simulink library "PowerFlowLib"  (R2016a)
settings: Solver=ode45  StartTime=0.0  StopTime=10.0  RelTol=1e-3
undefined symbols (not defined in the file or in its folder): Air, AirProp, C, F1, F2, Fanmap, Fld1, Fld2, Fluid, fueltankdata, HydProp, HydraulicLoad, IBFD_exc, L, LoadFluidProps, magnitude, MSSN, n_alghts, PumpProp, pwr_alghts, R_fd_exc, Rcore, Ts, VBFD_exc
libraries: PowerFlowLib x35, simulink x19, powerlib_extras x2, dspstat3 x2
(part 5 of 12)

== system PowerFlowLib/Energy & Power Systems/Electrical/Machines ==
  note: Electric Machines
  DC Position Servo : Subsystem  mask{Vf=390, Ra=0.5, La=0.9e-3, Rfsh=400, Lfsh=320, Lmsh=1.9, J=1.5, Ki=0.1}
      mask prompts: Vf "Field voltage (V)"; Ra "Armature resistance (Ohms)"; La "Armature inductance (H)"; Rfsh "Shunt field resistance (Ohms)"; Lfsh "Shunt field inductance (H)"; Lmsh "Mutual inductance (H)"; J "Rotor moment of inertia (Kgm^2)"; Ki "Integral constant for position loop (Ki)"
  DC Speed Servo : Subsystem  mask{Vf=390, Ra=0.05, La=0.9e-3, Rfsh=400, Lfsh=320, Lmsh=1.9, J=1.5}
      mask prompts: Vf "Field voltage (V)"; Ra "Armature resistance (Ohms)"; La "Armature inductance (H)"; Rfsh "Shunt field resistance (Ohms)"; Lfsh "Shunt field inductance (H)"; Lmsh "Mutual inductance (H)"; J "Rotor moment of inertia (Kgm^2)"
  Induction motor : Subsystem
      mask help: Induction Motor Model.
      mask init:
      | IM_fan_omega=[0;52.36;104.72;157.08;188.50;209.44;261.80;314.16;366.52;...
      |       376.99;418.88;471.24;523.60;565.49;575.96;628.32;680.68;733.04];
      | IM_fan_torque=[0;0.363;0.561;0.603;0.614;0.621;0.683;0.868;0.950;0.992;...
      |       1.134;1.269;1.460;1.700;1.750;2.044;2.262;2.618];
      |   
      | IM_wb=2*pi*200;  %base frequency
      | V_rated=132.8;  %rated phase voltage
      | IM_Lpr=114e-6; %Referred rotor leakage inductance
      | IM_Ls=114e-6;  %Stator leakage inductance
      | IM_Lm=0.0036;  %Magnetizing inductance
      | IM_rs=.0248; %Stator series resistance
      | IM_rrp=.01438; %referred rotor series resistance
      | IM_Xplr=IM_wb*IM_Lpr; %referred rotor leakage reactance
      | IM_Xls=IM_wb*IM_Ls;  %stator leakage reactance
      | IM_Xm=IM_wb*IM_Lm; %Magnetizing reactance
      | 
      | IM_Xr=IM_Xm+IM_Xplr;
      | IM_Xs=IM_Xm+IM_Xls;
      | IM_XM=1/(1/IM_Xm+1/IM_Xls+1/IM_Xplr);
      | IM_Lsp=1/IM_wb*(IM_Xls-IM_Xm^2/IM_Xplr);
      | IM_LR = IM_Lpr+IM_Lm;
      | IM_LS = IM_Ls+IM_Lm;
      | 
      | IM_Poles = 4;
      mask Display:
      | p1 = 0:0.1:(2*pi+0.1);
      | plot(sin(p1), cos(p1));
      | plot(0.8*sin(p1), 0.8*cos(p1));
      | plot(0.7*sin(p1), 0.7*cos(p1));
      | plot(0.3*sin(p1), 0.3*cos(p1));
      | p2 = 0:(pi/8):(2*pi);
      | for i = 1:length(p2);
      |     plot(0.05*sin(p1)+0.6*sin(p2(i)), 0.05*cos(p1)+0.6*cos(p2(i)));
      | end
      | port_label('output',1,'T_em')
      | port_label('output',2,'iqs')
      | port_label('output',3,'ids')
      | port_label('output',4,'i0s')
      | port_label('input',1,'vqs')
      | port_label('input',2,'vds')
      | port_label('input',3,'v0s')
      | port_label('input',4,'wr_mech')
  Permanent Magnet Synchronous Generator1 : Subsystem
      mask help: Permanent Magnet Synchronous Machine Model.
      mask init:
      | data_PMSM = load('exciter.mat');
      |   
      | % Lls_pm=500e-6;
      | % Lq=1.6e-3+Lls_pm;
      | % Ld=1e-3+Lls_pm;
      | Lls_pm = 5e-3;
      | Ld = data_PMSM.r(2);
      | Lq = data_PMSM.r(3);
      | Jm=data_PMSM.r(6);
      | l_m=data_PMSM.r(4);
      | Rs_pm=data_PMSM.r(1);
      | Poles = data_PMSM.r(5);
      | R_conv_exciter = 1/data_PMSM.r(7);
      | mc_exciter = data_PMSM.r(8);
      mask Display:
      | p1 = 0:0.1:(2*pi+0.1);
      | plot(sin(p1), cos(p1));
      | plot(0.8*sin(p1), 0.8*cos(p1));
      | plot(0.7*sin(p1), 0.7*cos(p1));
      | plot(0.3*sin(p1), 0.3*cos(p1));
      | plot([-0.2 0.2], [0.4 0.4], [0.2 0.3], [0.4 0.5], [-0.3 -0.2], [0.5 0.4]);
      | plot([-0.1 0.1], [0.6 0.6], [-0.1 0.1], [-0.6 -0.6], [0.6 0.6], [-0.1 0.1], [-0.6 -0.6], [-0.1 0.1]);
      | plot([0.4 0.4], [0.2 -0.2], [0.4 0.5], [0.2 0.3], [0.4 0.5], [-0.2 -0.3]);
      | plot([-0.2 0.2], [-0.4 -0.4], [0.2 0.3], [-0.4 -0.5], [-0.3 -0.2], [-0.5 -0.4]);
      | plot([-0.4 -0.4], [0.2 -0.2], [-0.4 -0.5], [0.2 0.3], [-0.4 -0.5], [-0.2 -0.3]);
      | port_label('output',1,'vqd0')
      | port_label('output',2,'Te')
      | port_label('output', 3, 'Ploss');
      | port_label('input',1,'iqd0')
      | port_label('input',2,'wr_m')
  Synchronous Machine P.U. dq0 : Subsystem  mask{machine_mode=20kVA_Gen}
      mask prompts: machine_mode "Machine Preset"
      mask help: Synchronous Machine p.u. Model in dq0 Frame.
      mask init:
      | switch machine_mode
      |     case 1
      |         preset = '20kVA_Gen.mat';
      |     case 2
      |         preset = '52.5kVA_Gen.mat';
      |     case 3
      |         preset = '100kVA_Gen.mat';
      |     case 4
      |         preset = '300kVA_Gen.mat';
      |     case 5
      |         preset = '800kVA_Gen.mat';
      |     otherwise
      |         preset = '1MVA_Gen.mat';
      | end
      | 
      | data = load(preset);
      | 
      | % Stator
      | Rs = data.r(1);
      | Xls = data.r(2);
      | Xmd = data.r(3);
      | Xmq = data.r(4);
      | 
      | % Field
      | R_fd = data.r(5);
      | Xlfd = data.r(6);
      | % Dampers
      | R_1d = data.r(7);
      | Xl1d = data.r(8);
      | R_1q = data.r(9);
      | Xl1q = data.r(10);
      | R_2q = data.r(11);
      | Xl2q = data.r(12);
      | 
      | % Rotor
      | P = data.r(13);
      | ws = data.r(14);
      | 
      | % Inductances
      | Xd = Xls + Xmd;
      | Xq = Xls + Xmq;
      | Xfd = Xlfd + Xmd;
      | X1q = Xl1q + Xmq;
      | Xd1 = Xd - Xmd^2/Xfd;
      | Xq1 = Xq - Xmq^2/X1q;
      | Xd2 = Xls + (1/(1/Xmd + 1/Xlfd + 1/Xl1d));
      | Xq2 = Xls + (1/(1/Xmq + 1/Xl1q + 1/Xl2q));
      | Tdo1 = Xfd/ws/R_fd;
      | Tqo1 = X1q/ws/R_1q;
      | Tdo2 = 1/ws/R_1d*(Xl1d + 1/(1/Xmd + 1/Xlfd));
      | Tqo2 = 1/ws/R_2q*(Xl2q+1/(1/Xmq + 1/Xl1q));
      | 
      | % Transmission Line
      | RTL = data.r(15);
      | XTL = data.r(16);
      | 
      | % Regulator and Governor
      | KA = data.r(17);
      | KF = data.r(18);
      | T_f = data.r(19);
      | TA = data.r(20);
      | KE = data.r(21);
      | TE = data.r(22);
      | 
      | % Base Quantities
      | SB = data.r(23);
      | VBDQ = data.r(24);
      | wB = data.r(25);
      | P = data.r(13);
      | H = data.r(26);
      | 
      | TB = (P/2)*SB/wB;
      | IBDQ = SB/VBDQ;
      | LBDQ = VBDQ/wB;
      | 
      | IBFD = IBDQ;
      | IB1D = IBDQ;
      | IB1Q = IBDQ;
      | IB2Q = IBDQ;
      | 
      | VBFD = SB/IBFD;
      | VB1D = SB/IB1D;
      | VB1Q = SB/IB1Q;
      | VB2Q = SB/IB2Q;
      | 
      | LBFD = VBFD/wB;
      | LB1D = VB1D/wB;
      | LB1Q = VB1Q/wB;
      | LB2Q = VB2Q/wB;
      | 
      | J = 2*data.r(26)/(wB*2/P)^2*SB;
      | M = 2*H/wB;
      | 
      | R_conv_gen = 1/data.r(27);
      | mc_gen = data.r(28);
      mask TypeOptions machine_mode: 20kVA_Gen | 52.5kVA_Gen | 100kVA_Gen | 300kVA_Gen | 800kVA_Gen | 1MVA_Gen
      mask Display:
      | p = 0:0.1:(2*pi+0.1);
      | plot(sin(p), cos(p));
      | p1 = (-pi/8-0.1-0.2):0.1:(pi/8+0.1-0.2);
      | plot(0.8*sin(p1), 0.8*cos(p1), 0.8*sin(p1+pi), 0.8*cos(p1+pi));
      | p2 = sin((-pi/8-0.1-0.2+pi/8+0.1-0.2)/2);
      | p3 = sin((-pi/8-0.1-0.2+pi/8+0.1-0.2)/2+pi);
      | p4 = cos((-pi/8-0.1-0.2+pi/8+0.1-0.2)/2);
      | p5 = cos((-pi/8-0.1-0.2+pi/8+0.1-0.2)/2+pi);
      | plot(0.8*[p2, p3], 0.8*[p4, p5]);
      | port_label('output', 1, 'Vdq0');
      | port_label('output', 2, 'Te');
      | port_label('output', 3, 'Vfd');
      | port_label('output', 4, 'Ploss');
      | port_label('input', 1, 'idq0');
      | port_label('input', 2, 'w');
      | port_label('input', 3, 'ifd');
  Transformer : Subsystem  mask(Transformer){Rp=0.005, Rs=0.1, N1=32, N2=355}
      mask prompts: Rp "Primary Winding Resistance"; Rs "Secondary Winding Resistance"; N1 "Number of Turns in Primary"; N2 "Number of Turns in Secondary"
      mask help:
      | The user inputs and outputs are given below. Inputs to the model are:
      |
      | Block Inputs
      | #1: Primary voltage input [V]
      | #2: Secondary current input [A]
      |
      | Block Outputs
      | #1: Secondary voltage output [V]
      | #2: Primary current input [A]
      mask Help: eval('open(''Transformer Help.html'')');
      mask Display:
      | image(imread('Transformer.png'))
      | 
      | port_label('input',1,'{\bf V_i_n}','TexMode','on')
      | port_label('input',2,'{\bf I_o_u_t}','TexMode','on')
      | 
      | port_label('output',1,'{\bf V_o_u_t}','TexMode','on')
      | port_label('output',2,'{\bf I_i_n}','TexMode','on')

== system PowerFlowLib/Energy & Power Systems/Electrical/Rectifiers ==
  note: Rectifier
  Single-phase Full Bridge Practical : Subsystem  mask(Single-phase full bridge rectifier.){C=100e-6, Rc=1}
      mask prompts: C "Output capacitance (F):"; Rc "Circuit parasitic resistance (ohm):"
      mask help: Single-phase Full bridge rectifier. Lead resistance is added to make simulation possible.
  Single-phase Half Bridge : Subsystem  mask(Single-phase half bridge rectifier.){C=100e-6, Rc=1}
      mask prompts: C "Output capacitance (F):"; Rc "Circuit parasitic resistance (ohm):"
      mask help: Single-phase half bridge rectifier. Lead resistance is added to make simulation possible.
  Three Phase Full Bridge Practical : Subsystem  mask(Single-phase full bridge rectifier.){C=100e-6, Rc=1}
      mask prompts: C "Output capacitance (F):"; Rc "Circuit parasitic resistance (ohm):"
      mask help: Single-phase Full bridge rectifier. Lead resistance is added to make simulation possible.
  Three-phase Full Bridge1 : Subsystem  mask(Single-phase full bridge rectifier.){C=100e-6, Rc=1}
      mask prompts: C "Output capacitance (F):"; Rc "Circuit parasitic resistance (ohm):"
      mask help: Single-phase Full bridge rectifier. Lead resistance is added to make simulation possible.
  three-phase active rectifier : Subsystem
      mask help: 3 phase active rectifier
  three-phase active rectifier Voltage Mode : Subsystem  mask(Rectifier){L=1e-3, C=1e-4}
      mask prompts: L "Inductance"; C "Capacitance"
      mask help:
      | The rectifier block converts ac voltage to dc voltage, which interfaces with the rest of the DC system.
      | This is an active rectifier and it is modeled in the synchronous dq0 reference frame.
      | The active rectifier control algorithm is omitted and a simplified model is implemented.
      |
      | Block Inputs:
      |
      | #1: Input line voltage in the synchronous reference frame [V]
      | #2: Converter modulation depth. It is a number between 0 and 1
      | #3: Output dc voltage level [V]
      |
      | Block Outputs:
      |
      | #1: Output DC current level [A]
      | #2: Input line current in the synchronous reference frame  [A]
      mask Display:
      | image(imread('Rectifier.png'))
      | 
      | % Define inputs
      | 
      | port_label('input',1,'{\bf V_d_q_0}','Texmode','on')
      | port_label('input',2,'{\bf m}','Texmode','on')
      | port_label('input',3,'{\bf V_D_C}','Texmode','on')
      | 
      | % Define outputs
      | 
      | port_label('output',1,'{\bf I_D_C}','Texmode','on')
      | port_label('output',2,'{\bf I_d_q_0}','Texmode','on')

== system PowerFlowLib/Energy & Power Systems/Electrical/Systems ==
  2 stage Boost converter (CCM Steady State) : Subsystem  mask(Cascaded Boost Converter CCM){KP=5, KI=1, VREF1=120}
      mask prompts: KP "Proportional constant"; KI "Integral constant"; VREF1 "Enter Stage 1 reference voltage (V) (Between 100 V and 150 V)"
      mask help: Two stage Boost Converter operated in steady state with a PI controller for duty ratio
  AC Service Bus : Subsystem
      mask help: Service Bus Structure.
      mask Display:
      | image(imread('ACbus.png')) % Load image
      | 
      | % Define inputs
      | 
      | port_label('input',1,'{\bf Select}','Texmode','on')
      | port_label('input',2,'{\bf Supply #1}','Texmode','on')
      | port_label('input',3,'{\bf Supply #2}','Texmode','on')
      | port_label('input',4,'{\bf Load}','Texmode','on')
      | 
      | % Define outputs
      | 
      | port_label('output',1,'{\bf Bus Voltage}','Texmode','on')
      | port_label('output',2,'{\bf Supply #1 Current}','Texmode','on')
      | port_label('output',3,'{\bf Supply #2 Current}','Texmode','on')
  DC Service Bus : Subsystem  mask(DC Service Bus){}
      mask help: Service Bus
      mask Display:
      | image(imread('DCbus.png')) % Load image
      | 
      | % Define inputs
      | 
      | port_label('input',1,'{\bf Select}','Texmode','on')
      | port_label('input',2,'{\bf Supply #1}','Texmode','on')
      | port_label('input',3,'{\bf Supply #2}','Texmode','on')
      | port_label('input',4,'{\bf Load}','Texmode','on')
      | port_label('input',5,'{\bf Charge}','Texmode','on')
      | 
      | % Define outputs
      | 
      | port_label('output',1,'{\bf Bus Voltage}','Texmode','on')
      | port_label('output',2,'{\bf Supply #1 Current}','Texmode','on')
      | port_label('output',3,'{\bf Supply #2 Current}','Texmode','on')
  GND Service Bus : Subsystem
      mask help: Ground Supply.
      mask Display:
      | image(imread('GPU2.jpg')) % Load image
      | 
      | % Define inputs
      | 
      | port_label('input',1,'{\bf I_d_q_0}','Texmode','on')
      | 
      | % Define outputs
      | 
      | port_label('output',1,'{\bf V_d_q_0}','Texmode','on')
  Gearbox : Subsystem  mask(Gearbox){Gear_Ratio=0.5620, Gear_Efficiency=98}
      mask prompts: Gear_Ratio "Gear Ratio"; Gear_Efficiency "Efficiency [%]"
      mask help:
      | Captures the effect of gear ratio on output shaft speed and torque.
      |
      | Input 1: Speed input [RPM]
      | Input 2: Torque input [Nm]
      |
      | Output 1: Speed output [RPM]
      | Output 2: Torque output [Nm]
      |
      | To simulate multiple gear ratios, vector inputs can be used for Gear Ratio and Efficiency.  Block outputs will be vectored signals of the same order.
      | Speed output = Speed input x Gear Ratio
      mask Display:
      | image(imread('Gearbox.png')) % Load image
      | 
      | % Define inputs
      | 
      | port_label('input',1,'{\bf \omega_e_n_g}','Texmode','on')
      | port_label('input',2,'{\bf \tau_e_n_g}','Texmode','on')
      | 
      | % Define outputs
      | 
      | port_label('output',1,'{\bf \omega_s_h_a_f_t}','Texmode','on')
      | port_label('output',2,'{\bf \tau_s_h_a_f_t}','Texmode','on')
  Gen Bus w/ APU switch : Subsystem  mask{LOWVLIMIT=90, UPVLIMIT=250, bus_st=2}
      mask prompts: LOWVLIMIT "Low voltage limit for generator cut-off (V)"; UPVLIMIT "Upper voltage limit for generator cut-off (V)"; bus_st "Bus voltage monitoring interval (s)"
      mask help: Generator Bus Structure.
  Generation Unit Sync-Sync : Subsystem  mask{machine_mode=100kVA_Gen, Rs=0.0163, Xls=0.00054, Xmd=0.66176, Xmq=0.00099, R_fd=0.016, Xlfd=0.2092, R_1d=0.2047, Xl1d=0.6524, R_1q=0.0429, R_2q=0.0429, Xl1q=0.0639, Xl2q=0.0639, ws=377, RTL=0.001, XTL=0.1, KA=20, KF=0.063, T_f=0.35, TA=0.2, KE=1, TE=0.314, SB=100000, VBDQ=100, wB=377, P=6, H=0.1777, R_conv_gen=0.05, mc_gen=10000, Vnom=115, fan_load='init_fan_characteristics.mat', exciter_param='exciter.mat'}
      mask prompts: machine_mode "Machine Preset"; Rs "Stator Resistance [ohm]"; Xls "Stator Leakage Reactance [ohm]"; Xmd "Magnetizing Direct Axis Reactance [ohm]"; Xmq "Magnetizing Quadrature Axis Reactance [ohm]"; R_fd "Field Resistance [ohm]"; Xlfd "Field Leakage Reactance [ohm]"; R_1d "Transient Direct Axis Resistance [ohm]"; Xl1d "Transient Leakage Direct Axis Reactance [ohm]"; R_1q "Transient Quadrature Axis Resistance [ohm]"; R_2q "Subtransient Quadrature Axis Resistance [ohm]"; Xl1q "Transient Leakage Quadrature Axis Reactance [ohm]"; Xl2q "Subtransient Leakage Quadrature Axis Reactance [ohm]"; ws "Rotational Speed [rad/s]"; RTL "Resistance [ohm]"; XTL "Reactance [ohm]"; SB "Baes Complex Power [VA]"; VBDQ "Base Direct and Quadrature Axis Armature Voltage [V]"; wB "Base Electrical Frequency [rad/s]"; P "Number of Pole Pairs"; H "Shaft Inertia Constant [s]"; Vnom "Nominal Voltage [V]"; fan_load "Fan Load"; exciter_param "Exciter Machine Parameters"
      mask help:
      | A generator system block implements a generic power generation unit consisting of a gearbox, a synchronous generator, a synchronous exciter and exciter controls.
      | The generator size can be selected from the drop window below.
      | (For advanced-users) When the User-defined option is selected from the drop window, the generator parameters can be manually specified in the tabs below.
      |
      | Block Inputs:
      |
      | #1: Jet engine low pressure spool [RPM]
      | #2: Exciter system supply voltage [V]
      | #3: Synchronous reference frame line currents  [A]
      |
      | Block Output:
      |
      | #1: Synchronous reference frame line voltages [V]
      | #2: Exciter system supply current [A]
      | #3: Electromagnetic torque on the low pressure spool  [N-M]
      | #4: Heat rejected to the cooling system or ambient [W]
      mask init:
      | load(fan_load);
      | 
      | % Inductances
      | Xd = Xls + Xmd;
      | Xq = Xls + Xmq;
      | Xfd = Xlfd + Xmd;
      | X1q = Xl1q + Xmq;
      | Xd1 = Xd - Xmd^2/Xfd;
      | Xq1 = Xq - Xmq^2/X1q;
      | Xd2 = Xls + (1/(1/Xmd + 1/Xlfd + 1/Xl1d));
      | Xq2 = Xls + (1/(1/Xmq + 1/Xl1q + 1/Xl2q));
      | Tdo1 = Xfd/ws/R_fd;
      | Tqo1 = X1q/ws/R_1q;
      | Tdo2 = 1/ws/R_1d*(Xl1d + 1/(1/Xmd + 1/Xlfd));
      | Tqo2 = 1/ws/R_2q*(Xl2q+1/(1/Xmq + 1/Xl1q));
      | 
      | % Base Quantities
      | 
      | TB = (P/2)*SB/wB;
      | IBDQ = SB/VBDQ;
      | LBDQ = VBDQ/wB;
      | 
      | IBFD = IBDQ;
      | IB1D = IBDQ;
      | IB1Q = IBDQ;
      | IB2Q = IBDQ;
      | 
      | VBFD = SB/IBFD;
      | VB1D = SB/IB1D;
      | VB1Q = SB/IB1Q;
      | VB2Q = SB/IB2Q;
      | 
      | LBFD = VBFD/wB;
      | LB1D = VB1D/wB;
      | LB1Q = VB1Q/wB;
      | LB2Q = VB2Q/wB;
      | 
      | J = 2*H/(wB*2/P)^2*SB;
      | M = 2*H/wB;
      | 
      | % Exciter
      | 
      | data_exc = load(exciter_param);
      |   
      | % Stator
      | Rs_exc = data_exc.r(1);
      | Xls_exc = data_exc.r(2);
      | Xmd_exc = data_exc.r(3);
      | Xmq_exc = data_exc.r(4);
      | 
      | % Field
      | R_fd_exc = data_exc.r(5);
      | Xlfd_exc = data_exc.r(6);
      | % Dampers
      | R_1d_exc = data_exc.r(7);
      | Xl1d_exc = data_exc.r(8);
      | R_1q_exc = data_exc.r(9);
      | Xl1q_exc = data_exc.r(10);
      | R_2q_exc = data_exc.r(11);
      | Xl2q_exc = data_exc.r(12);
      | 
      | % Rotor
      | P_exc = data_exc.r(13);
      | ws_exc = data_exc.r(14);
      | 
      | % Inductances
      | Xd_exc = Xls_exc + Xmd_exc;
      | Xq_exc = Xls_exc + Xmq_exc;
      | Xfd_exc = Xlfd_exc + Xmd_exc;
      | X1q_exc = Xl1q_exc + Xmq_exc;
      | Xd1_exc = Xd_exc - Xmd_exc^2/Xfd_exc;
      | Xq1_exc = Xq_exc - Xmq_exc^2/X1q_exc;
      | Xd2_exc = Xls_exc + (1/(1/Xmd_exc + 1/Xlfd_exc + 1/Xl1d_exc));
      | Xq2_exc = Xls_exc + (1/(1/Xmq_exc + 1/Xl1q_exc + 1/Xl2q_exc));
      | Tdo1_exc = Xfd_exc/ws_exc/R_fd_exc;
      | Tqo1_exc = X1q_exc/ws_exc/R_1q_exc;
      | Tdo2_exc = 1/ws_exc/R_1d_exc*(Xl1d_exc + 1/(1/Xmd_exc + 1/Xlfd_exc));
      | Tqo2_exc = 1/ws_exc/R_2q_exc*(Xl2q_exc+1/(1/Xmq_exc + 1/Xl1q_exc));
      | 
      | % Transmission Line
      | RTL_exc = data_exc.r(15);
      | XTL_exc = data_exc.r(16);
      | 
      | % Regulator and Governor
      | KA_exc = data_exc.r(17);
      | KF_exc = data_exc.r(18);
      | T_f_exc = data_exc.r(19);
      | TA_exc = data_exc.r(20);
      | KE_exc = data_exc.r(21);
      | TE_exc = data_exc.r(22);
      | 
      | % Base Quantities
      | SB_exc = data_exc.r(23);
      | VBDQ_exc = data_exc.r(24);
      | wB_exc = data_exc.r(25);
      | P_exc = data_exc.r(13);
      | H_exc = data_exc.r(26);
      | 
      | TB_exc = (P/2)*SB_exc/wB_exc;
      | IBDQ_exc = SB_exc/VBDQ_exc;
      | LBDQ_exc = VBDQ_exc/wB_exc;
      | 
      | IBFD_exc = IBDQ_exc;
      | IB1D_exc = IBDQ_exc;
      | IB1Q_exc = IBDQ_exc;
      | IB2Q_exc = IBDQ_exc;
      | 
      | VBFD_exc = SB_exc/IBFD_exc;
      | VB1D_exc = SB_exc/IB1D_exc;
      | VB1Q_exc = SB_exc/IB1Q_exc;
      | VB2Q_exc = SB_exc/IB2Q_exc;
      | 
      | LBFD_exc = VBFD_exc/wB_exc;
      | LB1D_exc = VB1D_exc/wB_exc;
      | LB1Q_exc = VB1Q_exc/wB_exc;
      | LB2Q_exc = VB2Q_exc/wB_exc;
      | 
      | J_exc = 2*data_exc.r(26)/(wB_exc*2/P_exc)^2*SB_exc;
      | M_exc = 2*H_exc/wB_exc;
      | 
      | R_conv_gen_exc = 1/data_exc.r(27);
      | mc_gen_exc = data_exc.r(28);
      mask Help: eval('open(''Generator System_help.html'')');
      mask TypeOptions machine_mode: 20kVA_Gen | 52.5kVA_Gen | 100kVA_Gen | 300kVA_Gen | 800kVA_Gen | 1MVA_Gen | User-defined
      mask Callback machine_mode:
      | h=get_param(gcb,'handle');
      | hblock=get(h);
      | data=load('GenProp.mat');
      | 
      | if strcmp(hblock.machine_mode,'User-defined')==1;
      |     adv_warn=warndlg(sprintf('User-defined parameters may lead to an unstable build.'));
      | 
      |     % grabs current values of enabled GUI parameters
      |     mskenabl = get_param(gcb,'MaskEnables');
      |     mskenabl(1:size(mskenabl,1)) = {'on'};  % sets all parameters to enable
      |     set_param(gcb,'MaskEnables',mskenabl)
      | 
      | else
      |     % For each generator preset references a column from GenProp.mat
      |     if strcmp(hblock.machine_mode,'20kVA_Gen')==1; n=1;
      |     elseif strcmp(hblock.machine_mode,'52.5kVA_Gen')==1; n=2;
      |     elseif strcmp(hblock.machine_mode,'100kVA_Gen')==1; n=3;
      |     elseif strcmp(hblock.machine_mode,'300kVA_Gen')==1; n=4;
      |     elseif strcmp(hblock.machine_mode,'800kVA_Gen')==1; n=5;
      |     elseif strcmp(hblock.machine_mode,'1MVA_Gen')==1; n=6;
      |     end
      |     % Set each parameter of the generator
      |     set1=num2str(data.r(1,n));
      |     set2=num2str(data.r(2,n));
      |     set3=num2str(data.r(3,n));
      |     set4=num2str(data.r(4,n));
      |     set_param(gcb,'Rs',set1,'Xls',set2,'Xmd',set3,'Xmq',set4)
      |     set1=num2str(data.r(5,n));
      |     set2=num2str(data.r(6,n));
      |     set_param(gcb,'R_fd',set1,'Xlfd',set2) %5 and 6
      |     set1=num2str(data.r(7,n));
      |     set2=num2str(data.r(8,n));
      |     set3=num2str(data.r(9,n));
      |     set4=num2str(data.r(10,n));
      |     set5=num2str(data.r(11,n));
      |     set6=num2str(data.r(12,n));
      |     set_param(gcb,'R_1d',set1,'Xl1d',set2,'R_1q',set3,'Xl1q',set4,'R_2q',set5,'Xl2q',set6) %7-12
      |     set1=num2str(data.r(14,n));
      |     set2=num2str(data.r(15,n));
      |     set3=num2str(data.r(16,n));
      |     set_param(gcb,'ws',set1,'RTL',set2,'XTL',set3)
      |     set1=num2str(data.r(17,n));
      |     set2=num2str(data.r(18,n));
      |     set3=num2str(data.r(19,n));
      |     set4=num2str(data.r(20,n));
      |     set5=num2str(data.r(21,n));
      |     set6=num2str(data.r(22,n));
      |     set_param(gcb,'KA',set1,'KF',set2,'T_f',set3,'TA',set4,'KE',set5,'TE',set6)
      |     set1=num2str(data.r(23,n));
      |     set2=num2str(data.r(24,n));
      |     set3=num2str(data.r(25,n));
      |     set4=num2str(data.r(13,n));
      |     set5=num2str(data.r(26,n));
      |     set_param(gcb,'SB',set1,'VBDQ',set2,'wB',set3,'P',set4,'H',set5)
      |     set1=num2str(1/data.r(27,n));
      |     set2=num2str(data.r(28,n));
      |     set_param(gcb,'R_conv_gen',set1,'mc_gen',set2)
      | 
      |     % grabs current values of enabled GUI parameters
      |     mskenabl = get_param(gcb,'MaskEnables');
      |     % sets all parameters to enable
      |     mskenabl(2:size(mskenabl,1)-3) = {'off'};
      |     set_param(gcb,'MaskEnables',mskenabl)
      | 
      | 
      | end
      | 
      | 
      | clear h hblock n data mskenabl
      | clear set1 set2 set3 set4 set5 set6
      mask Display:
      | image(imread('Generator.png')) % Load image
      | 
      | % Define inputs
      | 
      | port_label('input',1,'{\bf \omega_s_h_a_f_t}','Texmode','on')
      | port_label('input',2,'{\bf V_D_C}','Texmode','on')
      | port_label('input',3,'{\bf I_d_q_0}','Texmode','on')
      | port_label('input',4,'{\bf Temp}','Texmode','on')
      | 
      | % Define outputs
      | 
      | port_label('output',1,'{\bf V_d_q_0}','Texmode','on')
      | port_label('output',2,'{\bf I_D_C}','Texmode','on')
      | port_label('output',3,'{\bf \tau}','Texmode','on')
      | port_label('output',4,'{\bf P_l_o_s_s}','Texmode','on')
      | 
      | % % Define inputs
      | %
      | % port_label('input',1,'{\bf Generator Speed}','Texmode','on')
      | % port_label('input',2,'{\bf Battery Voltage}','Texmode','on')
      | % port_label('input',3,'{\bf Line Currents}','Texmode','on')
      | %
      | % % Define outputs
      | %
      | % port_label('output',1,'{\bf Line Voltages}','Texmode','on')
      | % port_label('output',2,'{\bf Battery Current}','Texmode','on')
      | % port_label('output',3,'{\bf Generator Torque}','Texmode','on')
      | % port_label('output',4,'{\bf Power Loss}','Texmode','on')
  Generator Bus : Subsystem
      mask help: Generator Bus Structure.
  Inverter Phase Control : Subsystem
      mask help: Inverter PWM Current Controller.
  Transformer-rectifier : Subsystem  mask{pu=1}
      mask prompts: pu "Voltage Regulation Level (p.u.)"
      mask Display:
      | image('TRU.png')
      | % Define Inputs
      | port_label('input',1,'{\bf V_d_q_0}','Texmode','on')
      | port_label('input',2,'{\bf V_D_C}','Texmode','on')
      | 
      | % Define Outputs
      | port_label('output',1,'{\bf I_D_C}','Texmode','on')
      | port_label('output',2,'{\bf I_d_q_0}','Texmode','on')
      | 
      | 
      | % % Define Inputs
      | % port_label('input',1,'{\bf Line Voltage}','Texmode','on')
      | % port_label('input',2,'{\bf Line Voltage}','Texmode','on')
      | %
      | % % Define Outputs
      | % port_label('output',1,'{\bf Line Voltage}','Texmode','on')
      | % port_label('output',2,'{\bf Line Voltage}','Texmode','on')
  three-phase full-bridge inverter : Subsystem
      mask help: Inverter

== system PowerFlowLib/Energy & Power Systems/Hydraulic/Bypass Valve ==
  Fluid In : Inport
  Req Flow : Inport  Port=2
  Bus Creator : BusCreator  Inputs=2
  Bus Creator1 : BusCreator  Inputs=3
  Bus Selector1 : BusSelector  OutputSignals=pres_kPa,temp_K,mdot_kgps
  Gain : Gain
  Gain1 : Gain
  Subtract : Sum  Inputs=+-
  Sum of Elements : Sum  Inputs=+
  Fluid Out : Outport
  Bypass : Outport  Port=2
  wires:
  Fluid In/1 -> Bus Selector1/1
  Bus Selector1/3 -> Subtract/1  "<mdot_kgps>"
  Req Flow/1 -> Sum of Elements/1
  Bus Creator/1 -> Fluid Out/1
  Bus Selector1/1 -> Bus Creator/1, Gain1/1  "<pres_kPa>"
  Bus Selector1/2 -> Bus Creator/2, Gain/1  "<temp_K>"
  Bus Creator1/1 -> Bypass/1
  Subtract/1 -> Bus Creator1/3  "mdot_kgps"
  Gain/1 -> Bus Creator1/2  "temp_K"
  Gain1/1 -> Bus Creator1/1  "pres_kPa"
  Sum of Elements/1 -> Subtract/2

== system PowerFlowLib/Energy & Power Systems/Hydraulic/Engine Driven Pump ==
  Fluid In : Inport
  Shaft RPM : Inport  Port=2
  Sys. Pres : Inport  Port=3
  Bus Creator : BusCreator  Inputs=3
  Bus Selector2 : BusSelector  OutputSignals=temp_K,pres_kPa
  Constant1 : Constant  Value=disp
  Constant4 : Constant  Value=nom_T + 273.15
  Constant5 : Constant  Value=eta_mech/100
  Constant6 : Constant  Value="nom_w / (2*pi) * disp * 1/100^3 * (1 - eta_v/100)  / nom_delP"
  Divide{2..3,5..6} (4 alike) : Product  Inputs=**
  Divide4 : Product  Inputs=*/
  Divide7 : Product  Inputs=*//*
  Gain : Gain
  RPS : Gain  Gain=1/60
  Sum1 : Sum  Inputs=|+-
  Sum2 : Sum  Inputs=|-+
  convert : Gain  Gain=1/100^3
  convert1 : Gain  Gain=2*pi
  convert2 : Gain  Gain=1000
  rho(T) : Lookup_n-D  NumberOfTableDimensions=1  BreakpointsForDimension1=HydProp.T  Table=HydProp.rho_T  RndMeth=Simplest  InputSameDT=on
  v(T) : Lookup_n-D  NumberOfTableDimensions=1  BreakpointsForDimension1=HydProp.T  Table=HydProp.mu_T  RndMeth=Simplest  InputSameDT=on
  v(T)nom : Lookup_n-D  NumberOfTableDimensions=1  BreakpointsForDimension1=HydProp.T  Table=HydProp.mu_T  RndMeth=Simplest  InputSameDT=on
  Fluid Out : Outport
  Shaft Torque : Outport  Port=2
  wires:
  Fluid In/1 -> Bus Selector2/1
  Bus Selector2/1 -> Gain/1, v(T)/1, rho(T)/1  "<temp_K>"
  RPS/1 -> Divide2/1, convert1/1  "rev/s"
  Constant1/1 -> convert/1  "cm^3 / rev"
  rho(T)/1 -> [rho]  "kg/m^3"
  Bus Creator/1 -> Fluid Out/1
  Shaft RPM/1 -> RPS/1  "rev/min"
  Bus Selector2/2 -> Sum2/1  "<pres_kPa>"
  Sys. Pres/1 -> Bus Creator/2, Sum2/2  "pres_kPa"
  convert/1 -> Divide2/2  "m^3 / rev"
  Gain/1 -> Bus Creator/1  "temp_K"
  Divide2/1 -> Sum1/1
  Constant4/1 -> v(T)nom/1
  v(T)nom/1 -> Divide3/1  "dyn viscosity"
  Constant6/1 -> Divide3/2
  Divide3/1 -> Divide4/1  "kHP"
  v(T)/1 -> Divide4/2  "dynamic viscosity"
  Divide4/1 -> Divide5/1  "kleak"
  Sum2/1 -> Divide5/2, [del_P]  "delP"
  Divide5/1 -> Sum1/2
  Sum1/1 -> Divide6/1, Divide7/4  "Vol flow rate"
  [rho] -> Divide6/2
  Divide6/1 -> Bus Creator/3  "mdot_kgps"
  [del_P] -> convert2/1  "kPa"
  Constant5/1 -> Divide7/2
  Divide7/1 -> Shaft Torque/1  "Torq_Nm"
  convert2/1 -> Divide7/1  "Pa"
  convert1/1 -> Divide7/3  "rad/s"

== system PowerFlowLib/Energy & Power Systems/Hydraulic/Fluid Reservoir ==
  Bleed In : Inport
  Bypass Return : Inport  Port=2
  mdot_out : Inport  Port=3
  Return : Inport  Port=4
  Bleed Valve on/off : Switch  Criteria=u2 ~= 0  ZeroCross=off
  Bus Creator : BusCreator  Inputs=2
  Bus Creator1 : BusCreator  Inputs=3
  Bus Selector2 : BusSelector  OutputSignals=pres_kPa
  Bus Selector3 : BusSelector  OutputSignals=temp_K,mdot_kgps
  Bus Selector4 : BusSelector  OutputSignals=pres_kPa,mdot_kgps,temp_K
  Divide : Product  Inputs=****/
  Divide1 : Product  Inputs=**/
  Divide2 : Product  Inputs=/*
  Gain : Gain  Gain=1/1000
  Gain1 : Gain  Gain=pres_loss/100
  R_air : Constant  Value=286.9
  Relational Operator : RelationalOperator  OutDataTypeStr=boolean
  Sum : Sum  Inputs=++-
  Sum of Elements : Sum  Inputs=+
  Sum1 : Sum  Inputs=|+-
  Sum2 : Sum  Inputs=-+|
  Sum3 : Sum  Inputs=-+|
  Temp : Integrator  InitialCondition=T_init  LimitOutput=on  LowerSaturationLimit=eps
  Terminator : Terminator
  Z(T,P) : Lookup_n-D  BreakpointsForDimension1=AirProp.T2  BreakpointsForDimension2=AirProp.P2  Table=AirProp.Z  RndMeth=Simplest  InputSameDT=on
  air pres : Integrator  InitialCondition=P_init*1000
  mass : Integrator  InitialCondition=mass_init  LimitOutput=on  LowerSaturationLimit=eps
  mass flow off : Constant  Value=0
  mass flow off1 : Constant  Value=bleed_flowrate
  resevor volume : Constant  Value=res_vol
  rho(T) : Lookup_n-D  NumberOfTableDimensions=1  BreakpointsForDimension1=HydProp.T  Table=HydProp.rho_T  RndMeth=Simplest  InputSameDT=on
  Bleed Demnd : Outport
  Fluid Conditions : Outport  Port=2
  wires:
  Bypass Return/1 -> Bus Selector3/1
  Bus Selector3/2 -> Divide1/2, Sum/1  "<mdot_kgps>"
  mdot_out/1 -> Sum/3, Bus Creator1/3  "mdot_kgps"
  Sum/1 -> mass/1  "dm/dt"
  Bus Selector4/3 -> Z(T,P)/1, Divide/3  "<temp_K>"
  R_air/1 -> Divide/1
  Z(T,P)/1 -> Divide/4
  Divide/1 -> air pres/1
  air pres/1 -> Gain/1
  resevor volume/1 -> Sum1/1
  Sum1/1 -> Divide/5
  Gain/1 -> Z(T,P)/2, Bus Creator/2, Bus Creator1/1  "pres_kPa"
  Gain1/1 -> Bus Creator/1, Sum2/1  "mdot_kgps"
  Bus Creator/1 -> Bus Selector2/1
  Sum2/1 -> Divide/2  "dm/dt"
  Bus Selector4/2 -> Terminator/1  "<mdot_kgps>"
  Bleed Valve on/off/1 -> Sum2/2, Bleed Demnd/1, Gain1/1
  Bus Selector4/1 -> Relational Operator/2  "<pres_kPa>"
  Bus Selector2/1 -> Relational Operator/1  "<pres_kPa>"
  mass flow off/1 -> Bleed Valve on/off/1
  Relational Operator/1 -> [valve_cmd]
  [valve_cmd] -> Bleed Valve on/off/2
  Bus Creator1/1 -> Fluid Conditions/1
  mass/1 -> Divide2/2, Divide1/3
  Divide1/1 -> Temp/1
  Sum3/1 -> Divide1/1
  Temp/1 -> Sum3/1, rho(T)/1, Bus Creator1/2  "temp_K"
  Bus Selector3/1 -> Sum3/2  "<temp_K>"
  Return/1 -> Sum of Elements/1
  Sum of Elements/1 -> Sum/2
  rho(T)/1 -> Divide2/1
  Divide2/1 -> Sum1/2
  mass flow off1/1 -> Bleed Valve on/off/3
  Bleed In/1 -> Bus Selector4/1

== system PowerFlowLib/Energy & Power Systems/Hydraulic/Hydraulic Load ==
  Fluid In : Inport
  Flight Phase : Inport  Port=2
  Bus Creator : BusCreator  Inputs=3
  Bus Selector1 : BusSelector  OutputSignals=pres_kPa,temp_K
  Divide : Product  Inputs=**/
  Gain : Gain
  Gain1 : Gain
  MATLAB Function : MATLAB Function  TreatAsAtomicUnit=on
  Memory : Memory
  Reset Timer : Subsystem
  m_dot : Lookup_n-D  BreakpointsForDimension1=[1:12]  BreakpointsForDimension2=[0:14999]  Table=HydraulicLoad.B_737.rudder  RndMeth=Simplest  InputSameDT=on
  rho(T) : Lookup_n-D  NumberOfTableDimensions=1  BreakpointsForDimension1=HydProp.T  Table=HydProp.rho_T  RndMeth=Simplest  InputSameDT=on
  Return : Outport
  Power : Outport  Port=2
  wires:
  Bus Creator/1 -> Return/1
  Fluid In/1 -> Bus Selector1/1
  Bus Selector1/1 -> Gain1/1  "<pres_kPa>"
  Bus Selector1/2 -> rho(T)/1, Gain/1  "<temp_K>"
  Flight Phase/1 -> MATLAB Function/2(curr_phase), Memory/1
  Memory/1 -> MATLAB Function/1(prev_phase)
  MATLAB Function/2(y) -> Reset Timer/1(Reset)
  Reset Timer/1(Count) -> m_dot/2
  MATLAB Function/1(phase_id) -> m_dot/1
  m_dot/1 -> Bus Creator/1, Divide/1  "mdot_kgps"
  rho(T)/1 -> Divide/3
  Divide/1 -> Power/1
  Gain1/1 -> Bus Creator/2, Divide/2  "pres_kPa"
  Gain/1 -> Bus Creator/3  "temp_K"

== system PowerFlowLib/Energy & Power Systems/Thermal/Anti-Ice ==
  Cntrl : Inport
  External Define : Constant  Value=0
  Load : Constant  Value=0
  LoadBus : BusCreator  Inputs=1
  LoadSwitch : Switch  Criteria=u2 > Threshold  Threshold=0.5
  No Load : Constant  Value=0
  Switch1 : Switch  Criteria=u2 > Threshold  Threshold=0.5
  data_sink : PowerFlowLib/Support Functions//Tools/data_sink
  Demand : Outport
  wires:
  Cntrl/1 -> LoadSwitch/2
  External Define/1 -> Switch1/2
  Switch1/1 -> LoadSwitch/1
  LoadBus/1 -> Demand/1
  No Load/1 -> LoadSwitch/3
  Load/1 -> Switch1/3
  ? -> Switch1/1
  LoadSwitch/1 -> data_sink/1, LoadBus/1  "pwr_kW"

== system PowerFlowLib/Energy & Power Systems/Thermal/ECS ==
  ACM : Subsystem  mask(Air Cycle Machine){Tw_init_phx=34, C_wall_phx=60000, N_init=15000, Comp_r1=.05, Comp_r2=.15, m_comp=10, Turb_r1=.15, Turb_r2=.1, m_turb=10, eta_b=.995, Qr=42000, PTurb_r1=0.05, PTurb_r2=0.025, m_pturb=10, Shft_r=.05, m_shft=10, J_comp=0.069808, J_turb=0.083289, J_pturb=0.0083036, J_shaft=0.0125}
      mask prompts: Tw_init_phx "Initial Wall Temperature [°C]"; C_wall_phx "Wall Heat Capacitance [J/K]"; N_init "Initial Rotational Speed [RPM]"; Comp_r1 "Entrance Tip Radius [m]"; Comp_r2 "Exit Tip Radius [m]"; m_comp "Mass [kg]"; Turb_r1 "Entrance Tip Radius [m]"; Turb_r2 "Exit Tip Radius [m]"; m_turb "Mass [kg]"; eta_b "Burner Efficiency [~]"; Qr "Fuel Heat of Reaction [kJ/kg]"; PTurb_r1 "Entrance Tip Radius [m]"; PTurb_r2 "Exit Tip Radius [m]"; m_pturb "Mass [kg]"; Shft_r "Radius [m]"; m_shft "Mass [kg]"; J_comp "Compressor"; J_turb "Expansion Turbine"; J_pturb "Power Turbine"; J_shaft "ACM Shaft"
      mask help:
      | Simulates the time varying temperatures throughout a four-wheel air cycle machine.
      |
      | Input 1: Flow into the compressor
      | Input 2: Flow into the power turbine
      | Input 3: Flow through primary heat exchanger
      |
      | Output 1: Flow out of expansion turbine
      | Output 2: RPM of ACM shaft
      mask init:
      | load Fluids
      | eval(['Air = Fluid.Air;']);
      | 
      | J_comp = (3/10) * m_comp * (Comp_r2^5 - Comp_r1^5) / (Comp_r2^3 - Comp_r1^3);
      | set_param(gcb,'J_comp',num2str(J_comp));
      | 
      | J_turb = (3/10) * m_comp * (Turb_r1^5 - Turb_r2^5) / (Turb_r1^3 - Turb_r2^3);
      | set_param(gcb,'J_turb',num2str(J_turb));
      | 
      | J_pturb = (3/10) * m_comp * (PTurb_r1^5 - PTurb_r2^5) / (PTurb_r1^3 - PTurb_r2^3);
      | set_param(gcb,'J_pturb',num2str(J_pturb));
      | 
      | J_shaft = (1/2) * m_shft * Shft_r^2;
      | set_param(gcb,'J_shaft',num2str(J_shaft));
      | 
      | set_param([gcb,'/Primary Heat Exchanger'],'Tw_init',num2str(Tw_init_phx));
      | set_param([gcb,'/Primary Heat Exchanger'],'C_wall',num2str(C_wall_phx));
      mask Display:
      | image(imread('revBrayton.png'))
      | text(0.5,0.95,['{\bf Air Cycle Machine}'],'TexMode','on','horizontalAlignment', 'center')
      | 
      | port_label('input',1,'{ \bfFlow In [Comp.]}','texmode','on')
      | port_label('input',2,'{ \bfFlow In [Power Turb]}','texmode','on')
      | port_label('input',3,'{ \bfFlow In [3rd Stream]}','texmode','on')
      | port_label('output',1,'{ \bfFlow Out}','texmode','on')
      | port_label('output',2,'{ \bfRPM}','texmode','on')
  Air-Air HX : Subsystem  mask(Air-Air Heat Exchanger){L_hx=0.2, W_hx=0.2, H_hx=0.2, t_p=0.0008, K_p=167, cp_hx=883, m_cm=16, l_fin=.005, t_fin=0.0002, s_fin=0.0015, h_fin=0.0095, K_n=167, eta_f=0.8, T_cm_0=50}
      mask prompts: L_hx "Length of HX in the flow direction [m]"; W_hx "Width of HX [m]"; H_hx "Height of HX [m]"; t_p "HX plate thickness [m]"; K_p "Thermal conductivity of the plates [W/m.K]"; cp_hx "Specific heat of the HX material [J/kg.K]"; m_cm "Mass of HX [kg]"; l_fin "Fin length [m]"; t_fin "Fin thickness [m]"; s_fin "Fin free flow width [m]"; h_fin "Fin free flow height [m]"; K_n "Thermal conductivity of the fin material [W/m.K]"; eta_f "Fin efficiency"; T_cm_0 "Initial_HX_core_temp_[C]"
      mask help:
      | In most aircraft applications, air-air heat exchangers are employed in the Air-cycle machine (ACM).
      | For the present implementation, a dynamic 1-D lumped parameter model is employed for characterizing the heat exchanger for B737 applications.
      |
      | Block Inputs:
      |
      | #1: Ram air inflow bus [Kg/s] [K] [kPa]
      | #2: Bleed air inflow bus [Kg/s] [K] [kPa]
      |
      | Block Outputs:
      |
      | #1: Ram air outflow bus [Kg/s] [K] [kPa]
      | #2: Bleed air outflow bus [Kg/s] [K] [kPa]
      | #3: Misc. Data
      mask init:
      | load AirProp
      mask Help: eval('open(''Air-Air_HX_help.html'')');
      mask Display:
      | image(imread('plate_hx.png'))
      | 
      | port_label('input',1,'{ \bfFlow In (Hot)}','texmode','on')
      | port_label('input',2,'{ \bfFlow In (Cold)}','texmode','on');
      | 
      | port_label('output',1,'{\bfFlow Out (Hot)}','texmode','on')
      | port_label('output',2,'{\bfFlow Out (Cold)}','texmode','on')
      | port_label('output',3,'{\bfMisc. Data}','texmode','on')
  Cabin Zone : Subsystem  mask(Passenger Cabin){A_fuselage=320, V_cab=130.3, n_pass=176, L_shell=0.003, K_shell=200, L_insulation=0.02, K_insulation=0.1, L_coating=0.002, K_coating=0.1, Vdot_sa_pass=0.009438, q_pass=60, RAR=0.5, h_outside=1, h_inside=1}
      mask prompts: A_fuselage "Total fuselage area [m^2]"; V_cab "Total cabin volume [m^3]"; n_pass "Total number of passengers [-]"; L_shell "Shell thickness [m]"; K_shell "Shell thermal conductivity [W/m.K]"; L_insulation "Insulation thickness [m]"; K_insulation "Insulation thermal conductivity [W/m.K]"; L_coating "Coating thickness [m]"; K_coating "Coating thermal conductivity [W/m.K]"; Vdot_sa_pass "Required supply air per passenger [m^3/Sec.pass]"; q_pass "Sensible heat release per passenger [W/pass]"; RAR "Recirculation air ratio [-]"; h_outside "Outside convective HT coefficient [W/m^2.K]"; h_inside "Inside convective HT coefficient [W/m^2.K]"
      mask help:
      | The passenger cabin model is a 1-D (lumped parameter) model, whereby the properties of the air inside the cabin are considered as uniform throughout the cabin (no spatial dependence).
      | The pressure and the temperature inside the cabin are derived through the conservation of mass and energy inside the control volume (cabin).
      | The passengers inside the cabin are considered as the source of sensible heat.
      | The heat transfer due to radiation and due to kinetic heating is accounted through approximate heat transfer coefficients.
      |
      | Block Inputs:
      |
      | #1: Supply air inflow bus [Kg/s][K][kPa]
      | #2: Ambient temperature [K]
      | #3: Mach number
      | #4: Equipment thermal load [W]
      |
      | Block Outputs:
      |
      | #1: Supply air demand [Kg/s]
      | #2: Cabin conditions [K] [kPa]
      | #3: Return air conditions [Kg/s][K][kPa]
      mask init:
      | load AirProp
      mask Help: eval('open(''Cabin Help.html'')');
      mask Display:
      | image(imread('cabin.png'))
      | port_label('input',1,'{ \bfFlow In}','texmode','on')
      | port_label('input',2,'{ \bfAmbient Temp.}','texmode','on')
      | port_label('input',3,'{ \bfMach #}','texmode','on')
      | port_label('input',4,'{ \bfThermal Loads}','texmode','on')
      | 
      | 
      | port_label('output',1,'{\bfCabin Conditions}','texmode','on')
      | port_label('output',2,'{\bfReturn Air Conditions}','texmode','on')
  Cargo bay : Subsystem  mask(Cargo Bay){T_cargo_K=305}
      mask prompts: T_cargo_K "Desired Cargo temperature (K)"
      mask Display:
      | port_label('input',1,'{ \bfReturn Air Conditions}','texmode','on')
      | port_label('input',2,'{ \bfThermal Loads}','texmode','on')
      | port_label('input',3,'{ \bfFlow from Right PACK}','texmode','on')
      | 
      | 
      | port_label('output',1,'{\bfFlow Distributor}','texmode','on')
      | port_label('output',2,'{\bfCargo to fan}','texmode','on')
  Compressor : Subsystem
      mask help:
      | The turbocharger consists of a turbine driven by the exhaust gas and connected via a common shaft to the compressor, which compresses the air in the intake.
      | The rotational speed (N) of the turbocharger shaft can be derived as a power (P) balance between the turbine and the compressor side.
      |
      | Block Inputs:
      |
      | #1: Engine Bleed [Kg/s] [K] [kPa]
      | #2: Shaft Speed [W]
      |
      | Block Outputs:
      |
      | #1: Engine Bleed [Kg/s] [K] [kPa]
      | #2: Compressor Power [W]
      mask init:
      | load AirProp
      | load CompProp
      mask Help:
      | Main Assumptions
      | 1. The Turbine and the compressor are coupled to each other (turbocharger).
      | 2. Maps are provided to compute the efficiency of the compressor.
      | 3. There is no heat transfer from the compressor to the surrounding.
      mask Display:
      | image(imread('compressor.png'))
      | port_label('input',1,'{ \bfFlow In}','texmode','on')
      | port_label('input',2,'{ \bfShaft Speed}','texmode','on');
      | 
      | 
      | port_label('output',1,'{\bfFlow Out}','texmode','on')
      | port_label('output',2,'{\bfComp. Work}','texmode','on')
  Fan : Subsystem  mask(Fan){N_fan=1725}
      mask prompts: N_fan "Fan speed [rpm]"
      mask help:
      | The function of a fan in the ECS is to deliver the recirculated air from the cabin to a mixing junction, where the recirculated air is mixed with the conditioned air from the ECS.
      | The fan model in Simulink determines the recirculated air properties and the fan power required.
      |
      | Block Inputs:
      |
      | #1: Input flow bus [Kg/s] [K] [kPa]
      |
      | Block Outputs:
      |
      | #1: From cabin to fan  [Kg/s] [K] [kPa]
      | #2: Other output bus [RPM] [kW]
      mask init:
      | load AirProp
      | load Fanmap
      mask Help:
      | Main Assumptions:
      | 
      | 1. Fan performance data based on GREENHECK-SQ 130.
      | 2. Volume flow rate allowable operating range: 891 to 2368 cfm based
      | on the chosen performance data.
      | 3. Constant speed operation at 1725 rpm (the input rpm in the mask is only intended for future
      | upgrade of the fan model into a variable speed one).
      | 4. Air properties are calculated at inlet conditions.
      | 5. Outlet air temperature is based on heating by all the power loss
      mask Display:
      | image(imread('fan.png'))
      | 
      | port_label('input',1,'{ \bfFlow In}','texmode','on')
      | 
      | port_label('output',1,'{\bfFlow Out}','texmode','on')
      | port_label('output',2,'{\bfFan Data}','texmode','on')
  T_35_valve : Subsystem  mask{T_35=273}
      mask prompts: T_35 "Specify the temperature at this junction (K)."
      mask help: 35 F VALVE (ECS)
      mask Help:
      | Main Assumptions
      | 1. The valve regulates the flow rate such that the air temperature
      | downstream of the turbine is at 276 K.
      | 2. A map of the valve opening against the mass flow rate is provided
      | 3. The pressure drop across the valve is assumed to be zero.
      mask Display:
      | port_label('input',1,'{ \bfFlow bypass from P.HX}','texmode','on')
      | port_label('input',2,'{ \bfFlow monitor - T.exit}','texmode','on');
      | 
      | 
      | port_label('output',1,'{\bfFlow to Comp. }','texmode','on')
      | port_label('output',2,'{\bfTotal flow to Mix.junct }','texmode','on')
  Turbine : Subsystem  mask{press_Turbine_exit=80, inertia=5e-5, n_t=0.7}
      mask prompts: press_Turbine_exit "Turbine exit pressure (kPa)"; inertia "Turbine Inertia"; n_t "Turbine Efficiency"
      mask help:
      | The turbocharger consists of a turbine driven by the exhaust gas and connected via a common shaft to the compressor, which compresses the air in the intake.
      | The rotational speed (N) of the turbocharger shaft can be derived as a power (P) balance between the turbine and the compressor side.
      |
      | Block Inputs:
      |
      | #1: Engine Bleed [Kg/s] [K] [kPa]
      | #2: Compressor Power [W]
      |
      | Block Outputs:
      |
      | #1: Engine Bleed [Kg/s] [K] [kPa]
      | #2: Shaft Speed [RPM]
      | #3; Turbine Power[W]
      mask init:
      | load AirProp
      mask Help:
      | Main Assumptions
      | 1. The Turbine and the compressor are coupled to each other (turbocharger).
      | 2. The efficiency of the turbine is constant.
      | 3. There is no heat transfer from the turbine to the surrounding.
      | 4. The initial speed of the turbine should be non-zero (which simulates a starting torque).
      mask Display:
      | image(imread('turbine.png'))
      | 
      | port_label('input',2,'{ \bfComp. Work}','texmode','on')
      | port_label('input',1,'{ \bfFlow In}','texmode','on')
      | 
      | 
      | port_label('output',2,'{\bfShaft Speed}','texmode','on')
      | port_label('output',1,'{\bfFlow Out}','texmode','on')
      | port_label('output',3,'{\bfTurb. Work}','texmode','on')
  n-intlet Mixing Junction : Subsystem  mask(Mixing Junction){no_inlets=3, d_in_1=0.1, d_in_2=0.1, d_out=0.2}
      mask prompts: no_inlets "Number of Inlets (Max: 10)"; d_in_1 "Diameter of the inlet duct (1)"; d_in_2 "Diameter of the inlet duct (2)"; d_out "Diameter of the outlet duct"
      mask init:
      | load AirProp
      | 
      | h      = get_param(gcb,'handle');   % Get block handle
      | blk    = gcb; 
      | hblock = get(h);     % Parse out handles structure 
      | 
      | 
      | % set each vector concat to have n number of inputs
      | set_param([blk,'/temp_vector'],'NumInputs',hblock.no_inlets);
      | set_param([blk,'/pres_vector'],'NumInputs',hblock.no_inlets);
      | set_param([blk,'/mdot_vector'],'NumInputs',hblock.no_inlets);
      | 
      | % delete any previous inports and bus selectors
      | for i = str2num(hblock.no_inlets)+1:hblock.Ports(1)
      |    delete_block([blk,'/Inlet#',num2str(i)])
      |    delete_block([blk,'/BusSel#',num2str(i)])
      |    delete_unconnected_lines(blk)
      | end
      | 
      | % generate inports, bus selectors, and route lines to each vector concat
      | for i = hblock.Ports(1)+1:str2num(hblock.no_inlets)
      |     add_block('built-in/Inport',[blk,'/Inlet#',num2str(i)],'Position',[30 i*80-25 60 i*80-12]);         % adding inport
      |     add_block('built-in/BusSelector',[blk,'/BusSel#',num2str(i)],'Position',[75 80*i-50 80 80*i+10]);   % adding bus selector
      |     add_line(blk,['Inlet#',num2str(i),'/1'],['BusSel#',num2str(i),'/1']);                               % line added
      |     set_param([blk,'/BusSel#',num2str(i)],'OutputSignals','pres_kPa,temp_K,mdot_kgps')                  % setting bus signals
      |     add_line(blk,['BusSel#',num2str(i),'/1'],['pres_vector/',num2str(i)],'AutoRouting','on')
      |     add_line(blk,['BusSel#',num2str(i),'/2'],['temp_vector/',num2str(i)],'AutoRouting','on')
      |     add_line(blk,['BusSel#',num2str(i),'/3'],['mdot_vector/',num2str(i)],'AutoRouting','on')
      | end
      | 
      | clear h blk hblock
      mask Help: eval('open(''MixingJunction_help.html'')');
      mask Callback no_inlets:
      | h      = get_param(gcb,'handle');   % Get block handle
      | blk    = gcb;
      | hblock = get(h);     % Parse out handles structure
      | 
      | if str2num(hblock.no_inlets) > 10
      |     set_param(blk,'no_inlets',num2str(10))
      | end
      | 
      | clear h blk hblock
      mask Display:
      | image(imread('MergeImage.png'))
      | 
      | h      = get_param(gcb,'handle');   % Get block handle
      | blk    = gcb;
      | hblock = get(h);     % Parse out handles structure
      | 
      | for i = 1:str2num(hblock.no_inlets)
      |     port_label('input',i,['{\bf Inlet #',num2str(i),'}'],'TexMode','on')
      | 
      | end
      | 
      | port_label('output',1,'{\bf Flow Out}','texmode','on')
